simulink library "source_mod"  (R2019b)
settings: Solver=VariableStepAuto  StartTime=0.0  StopTime=10.0  RelTol=1e-3
undefined symbols (not defined in the file or in its folder): gcbh, sps_rtmsupport
libraries: spsSourcesModel x1
settings Model: Creator=josuegutierrezledesma  LastModifiedBy=Alejandro
settings DebuggingCC: ArithmeticOperatorsInVariantConditions=warning
settings SFSimCC: CustomCodeUndefinedFunction=UseInterfaceOnly

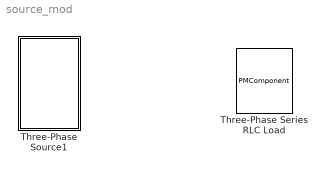
== system source_mod ==
  Three-Phase Series RLC Load : PMComponent  DialogController=POWERSYS.PowerSysDialog  LoadFcn=sps_rtmsupport('LoadFcn',gcbh);  StartFcn=sps_rtmsupport('StartFcn',gcbh);  StopFcn=sps_rtmsupport('StopFcn',gcbh);  PhysicalDomain=powersysdomain  LeftPortType=p1  RightPortType=p1  LConnTagsString=A|B|C  mask(Three-Phase Series RLC Load){Configuration=Y (grounded), NominalVoltage=1000, Vabc=[1e3 1e3 1e3], Vabcp=[1e3 1e3 1e3], NominalFrequency=60, UnbalancedPower=off, ActivePower=10e3, InductivePower=100, CapacitivePower=100, Pabc=[10e3 9e3 11e3], QLabc=[100 90 110], QCabc=[100 90 110], Pabcp=[10e3 9e3 11e3], QLabcp=[100 90 110], QCabcp=[100 90 110], Measurements=None, LoadType=constant Z}
      mask prompts: NominalVoltage "Nominal phase-to-phase voltage Vn (Vrms)"; Vabc "Nominal phase-to-neutral voltages [Va Vb Vc] (Vrms)"; Vabcp "Nominal phase-to-phase voltages [Vab Vbc Vca] (Vrms)"; NominalFrequency "Nominal frequency fn (Hz):"; UnbalancedPower "Specify PQ powers for each phase"; ActivePower "Active power P (W):"; InductivePower "Inductive reactive power QL (positive var):"; CapacitivePower "Capacitive reactive power Qc (negative var):"; Pabc "Active powers [Pa Pb Pc] (W):"; QLabc "Inductive reactive powers [QLa QLb QLc] (positive var):"; QCabc "Capacitive reactive powers [QCa QCb QCc] (negative var):"; Pabcp "Active powers [Pab Pbc Pca] (W):"; QLabcp "Inductive reactive powers [QLab QLbc QLca] (positive var):"; QCabcp "Capacitive reactive powers [QCab QCbc QCca] (negative var):"; LoadType "Load type:"
      mask help: Implements a three-phase series RLC load.
      mask init:
      | [s1,s2,s3,s4,r1,r2,l1,l2,c1,c2,c3,c4] = powericon('Series RLC Load',ActivePower,InductivePower,CapacitivePower,UnbalancedPower,Pabc,QLabc,QCabc,Pabcp,QLabcp,QCabcp,Configuration);
      | ground = Configuration==1;
      | neutral = Configuration==3;
      | power_initmask();
      settings: AttributesFormatString=\n  CopyFcn=sps_rtmsupport('CopyFcn',gcbh);  DeleteFcn=sps_rtmsupport('DeleteFcn',gcbh);  UndoDeleteFcn=sps_rtmsupport('UndoDeleteFcn',gcbh);  ModelCloseFcn=sps_rtmsupport('ModelCloseFcn',gcbh);  PreSaveFcn=sps_rtmsupport('PreSaveFcn',gcbh);  PostSaveFcn=sps_rtmsupport('PostSaveFcn',gcbh);  NameChangeFcn=sps_rtmsupport('NameChangeFcn',gcbh);  PreCopyFcn=sps_rtmsupport('PreCopyFcn',gcbh);  OpenFcn=sps_rtmsupport('OpenFcn',gcbh, [1 6 16 17]);  CloseFcn=sps_rtmsupport('CloseFcn',gcbh);  PreDeleteFcn=sps_rtmsupport('PreDeleteFcn',gcbh);
      mask Help: helpview(psbhelp);
      mask TypeOptions Configuration: Y (grounded) | Y (floating) | Y (neutral) | Delta
      mask Callback Configuration: powericon('ThreePhaseLoadBlocksCback',gcb);
      mask Callback UnbalancedPower: powericon('ThreePhaseLoadBlocksCback',gcb);
      mask TypeOptions Measurements: None | Branch voltages | Branch currents | Branch voltages and currents
      mask TypeOptions LoadType: constant Z | constant PQ | constant I
      mask DialogControl Parameters Prompt: Parameters
      mask DialogControl LoadFlow Prompt: Load Flow
      mask Display:
      | plot(s1-60,s2,s3+80,s4,r1,r2,l1,l2,c1,c2,c3,c4)
      | 
      | plot( ground*[s3,s3], ground*[-s2/4,s2/4])
      | plot( ground*[s3+30,s3+30], ground*[-s2/6,s2/6])
      | plot( ground*[s3+60,s3+60], ground*[-s2/10,s2/10])
      | 
      | plot( neutral*[s3,s3+80], neutral*[0,0])
      | 
      | port_label('LConn', 1, 'A')
      | port_label('LConn', 2, 'B')
      | port_label('LConn', 3, 'C')
  Three-Phase Source1 : Subsystem  DialogController=POWERSYS.PowerSysDialog  LoadFcn=sps_rtmsupport('LoadFcn',gcbh);  StartFcn=sps_rtmsupport('StartFcn',gcbh);  StopFcn=sps_rtmsupport('StopFcn',gcbh);  mask(Three-Phase Source){InternalConnection=Yg, VoltagePhases=off, Voltage=0, PhaseAngle=0, Voltage_phases=[25e3 25e3 25e3]/sqrt(3), PhaseAngles_phases=[0 -120 +120], Frequency=50, NonIdealSource=off, SpecifyImpedance=on, Resistance=0.8929, Inductance=16.58e-3, ShortCircuitLevel=100e6, BaseVoltage=69e3, XRratio=7, BusType=PV, Pref=40e6, Qref=0, Prefabc=[10e3, 10e3, 10e3], Qrefabc=[0, 0, 0], Qmin=-40e6, Qmax=50e6}
      mask prompts: InternalConnection "Configuration:"; VoltagePhases "Specify internal voltages for each phase"; Voltage "Phase-to-phase voltage (Vrms):"; PhaseAngle "Phase angle of phase A (degrees):"; Voltage_phases "Line-to-neutral voltages [Va Vb Vc] (Vrms)"; PhaseAngles_phases "Phase angle of line-to-neutral voltages [phia phib phic] (deg)"; Frequency "Frequency (Hz):"; NonIdealSource "Internal"; SpecifyImpedance "Specify short-circuit level parameters"; Resistance "Source resistance (Ohms):"; Inductance "Source inductance (H):"; ShortCircuitLevel "3-phase short-circuit level at base voltage(VA):"; BaseVoltage "Base voltage (Vrms ph-ph):"; XRratio "X/R ratio:"; BusType "Generator type:"; Pref "Active power generation P (W)"; Qref "Reactive power generation Q (var)"; Prefabc "Active power generation [Pa Pb Pc] (W)"; Qrefabc "Reactive power generation [Qa Qb Qc] (var)"; Qmin "Minimum reactive power Qmin or [Qamin,Qbmin Qcmin] (var)"; Qmax "Maximum reactive power Qmax or [Qamax,Qbmax Qcmax] (var)"
      mask help: Three-phase voltage source in series with RL branch.
      mask init:
      | block = gcb;
      | powericon('ThreePhaseSourceCback',block);
      | [s1,s2,s3,s4,g1,g2,g3,g4,g5,g6,s5] = powericon('ThreePhaseSourceIcon',SpecifyImpedance,ShortCircuitLevel,BaseVoltage,Resistance,Inductance,XRratio,InternalConnection,NonIdealSource);
      | powericon('psbloadfunction',block,'goto','Initialize');
      | [Ts, WantBlockChoice,Aa,Pa,Ab,Pb,Ac,Pc] = powericon('ThreePhaseSourceInit',block,Voltage,PhaseAngle,Voltage_phases,PhaseAngles_phases,VoltagePhases);
      | powericon('SetInternalModels','set',block,WantBlockChoice);
      settings: CopyFcn=sps_rtmsupport('CopyFcn',gcbh); powericon('psbloadfunction',gcb,'goto','UpdateGotoTag');  DeleteFcn=sps_rtmsupport('DeleteFcn',gcbh);  UndoDeleteFcn=sps_rtmsupport('UndoDeleteFcn',gcbh);  ModelCloseFcn=sps_rtmsupport('ModelCloseFcn',gcbh);  PreSaveFcn=sps_rtmsupport('PreSaveFcn',gcbh);  PostSaveFcn=sps_rtmsupport('PostSaveFcn',gcbh);  NameChangeFcn=sps_rtmsupport('NameChangeFcn',gcbh);  PreCopyFcn=sps_rtmsupport('PreCopyFcn',gcbh);  OpenFcn=sps_rtmsupport('OpenFcn',gcbh, [1,2,8,-9,15]);  CloseFcn=sps_rtmsupport('CloseFcn',gcbh);  PreDeleteFcn=sps_rtmsupport('PreDeleteFcn',gcbh);
      mask Help: helpview(psbhelp);
      mask TypeOptions InternalConnection: Y | Yn | Yg
      mask Callback InternalConnection: %powericon('ThreePhaseSourceCback',gcb);
      mask Callback VoltagePhases: powericon('ThreePhaseSourceCback',gcb);
      mask Callback NonIdealSource: powericon('ThreePhaseSourceCback',gcb);
      mask Callback SpecifyImpedance: powericon('ThreePhaseSourceCback',gcb);
      mask TypeOptions BusType: swing | PV | PQ
      mask Callback BusType: powericon('ThreePhaseSourceCback',gcb);
      mask Callback Qmax: sps_rtmsupport('parametereditingmodes',gcbh, [1,2,8,-9,15]);
      mask DialogControl Parameters Prompt: Parameters
      mask DialogControl Container7 Prompt: Source
      mask DialogControl Container6 Prompt: Impedance
      mask DialogControl LoadFlow Prompt: Load Flow
      mask Display:
      | plot(-180,-50,s5,50,s1,s2,s3,s4,[0,9,18,24,29,30,29,24,18,9,0,-9,-18,-24,-29,-30,-29,-24,-18,-9,0]*1.5-45, [30,29,24,18,9,0,-9,-18,-24,-29,-30,-29,-24,-18,-9,0,9,18,24,29,30]*0.8,[-150,-90],[0,0]);
      | plot(g1,g2,g3,g4,g5,g6);
      | plot([1 2 3 4 5 6 7 8 9 10 11 12 13 14 15 16 17 18 19 20 21].*2.5-72, [0,9,18,24,29,30,29,24,18,9,0,-9,-18,-24,-29,-30,-29,-24,-18,-9,0]./3)

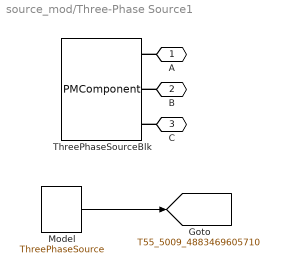
== system source_mod/Three-Phase Source1 ==
  Model : spsSourcesModel/ThreePhaseSource  SystemSampleTime=-1  Latency=0  AutoFrameSizeCalculation=off
      settings: SourceProductName=Simscape Electrical  SourceProductBaseCode=PS
  ThreePhaseSourceBlk : PMComponent  PhysicalDomain=powersysdomain  LeftPortType=p1  RightPortType=p1  LConnTagsString=N  RConnTagsString=A|B|C  mask(InnerPowersysBlock){}
      mask Display: disp('SPS internal use\nDo not delete')
  A : PMIOPort  Side=Right
  B : PMIOPort  Port=2  Side=Right
  C : PMIOPort  Port=3  Side=Right
  tag scope: T55_5009_4883469605710=global
  wires:
  Model/1 -> [T55_5009_4883469605710]
  connections:
  C/RConn1 -- ThreePhaseSourceBlk/RConn3
  B/RConn1 -- ThreePhaseSourceBlk/RConn2
  A/RConn1 -- ThreePhaseSourceBlk/RConn1
